simulink subsystem "Command_Data_handling"  (R2024a)
settings: Solver=VariableStepAuto  StartTime=0.0  StopTime=10.0  RelTol=1e-3
undefined symbols (not defined in the file): rfSatSourceSampleTime
libraries: simulink x1, commrandsrc3 x1
settings Model: Creator=dani  LastModifiedBy=dani

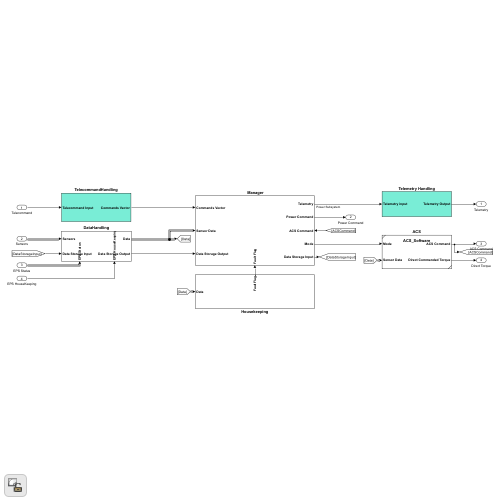
[thumbnail: Simulink's stored preview of the top-level diagram]
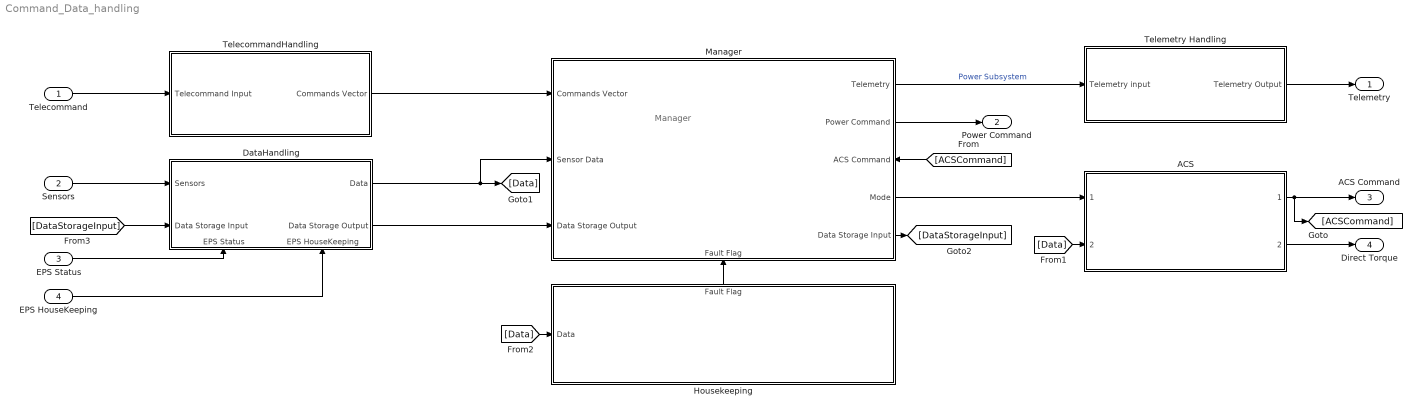
== system Command_Data_handling ==
  note: Manager
  Telecommand : Inport
  Sensors : Inport  Port=2
  EPS Status : Inport  Port=3
  EPS HouseKeeping : Inport  Port=4
  " Manager" : Subsystem
      settings: PortSchema="{\"entries\":[{\"content\":{\"sides\":[{\"content\":{\"connectorIds\":[\"In1\",\"In2\",\"In3\"]},\"type\":\"ConnectorPlacement.EquallySpacedRectSide\",\"uuid\":\"ec07d368-8191-42e4-9375-c2c602df22cf\"},{\"content\":{\"connectorIds\":[\"Out1\",\"Out2\",\"In5\",\"Out3\",\"Out4\"],\"side\":\"RIGHT\"},\"type\":\"ConnectorPlacement.EquallySpacedRectSide\",\"uuid\":\"bfabc2f5-2100-4bb6-919b-28e5c4a4cd4f\"},{\"content\":{\"side\":\"TOP\"},\"type\":\"ConnectorPlacement.EquallySpacedRectSide\",\"uuid\":\"1116e096-0190-44f1-9e3d-e2304f4178f6\"},{\"content\":{\"connectorIds\":[\"In4\"],\"side\":\"BOTTOM\"},\"type\":\"ConnectorPlacement.EquallySpacedRectSide\",\"uuid\":\"3d921d5d-5d93-4419-baa2-2f36ac6a4a99\"}]},\"type\":\"ConnectorPlacement.EquallySpacedConnector\",\"uuid\":\"03acd5cc-f7c7-46e5-a21e-c8fb7c082571\"}],\"packageUris\":[\"http://schema.mathworks.com/mf0/Connector/R2020b\"],\"version\":\"1.0\"}"
  ACS : Subsystem  ReferencedSubsystem=ACS_Software
  DataHandling : Subsystem
      settings: PortSchema="{\"entries\":[{\"content\":{\"sides\":[{\"content\":{\"connectorIds\":[\"In1\",\"In2\"]},\"type\":\"ConnectorPlacement.EquallySpacedRectSide\",\"uuid\":\"333a63f6-0788-485d-a40f-b2eefd028988\"},{\"content\":{\"connectorIds\":[\"Out1\",\"Out2\"],\"side\":\"RIGHT\"},\"type\":\"ConnectorPlacement.EquallySpacedRectSide\",\"uuid\":\"78b8a504-3dff-4f2b-a0ec-fa2bfb715213\"},{\"content\":{\"side\":\"TOP\"},\"type\":\"ConnectorPlacement.EquallySpacedRectSide\",\"uuid\":\"ac4bbea7-d5e7-4844-aab9-f621cfd7c534\"},{\"content\":{\"connectorIds\":[\"In3\",\"In4\"],\"side\":\"BOTTOM\"},\"type\":\"ConnectorPlacement.EquallySpacedRectSide\",\"uuid\":\"8bcb476b-069e-40da-9a40-a3d9d3480925\"}]},\"type\":\"ConnectorPlacement.EquallySpacedConnector\",\"uuid\":\"bbb35b76-fa73-457a-a216-c7062a4ce149\"}],\"packageUris\":[\"http://schema.mathworks.com/mf0/Connector/R2020b\"],\"version\":\"1.0\"}"
  Housekeeping : Subsystem
      settings: PortSchema="{\"entries\":[{\"content\":{\"sides\":[{\"content\":{\"connectorIds\":[\"In1\"]},\"type\":\"ConnectorPlacement.EquallySpacedRectSide\",\"uuid\":\"8eabc5dd-b460-4602-97d0-241e39b04916\"},{\"content\":{\"side\":\"RIGHT\"},\"type\":\"ConnectorPlacement.EquallySpacedRectSide\",\"uuid\":\"34fc1683-6b23-42e6-b522-0d805f5ee3a0\"},{\"content\":{\"connectorIds\":[\"Out1\"],\"side\":\"TOP\"},\"type\":\"ConnectorPlacement.EquallySpacedRectSide\",\"uuid\":\"2e5f843e-dd0f-45a3-97ce-c55e6bc4c9fd\"}]},\"type\":\"ConnectorPlacement.EquallySpacedConnector\",\"uuid\":\"4787b5c4-2ae8-477e-a21f-abe35d36bbd4\"}],\"packageUris\":[\"http://schema.mathworks.com/mf0/Connector/R2020b\"],\"version\":\"1.0\"}"
  TelecommandHandling : Subsystem
  Telemetry Handling : Subsystem
  Telemetry : Outport
  Power Command : Outport  Port=2
  ACS Command : Outport  Port=3
  Direct Torque : Outport  Port=4
  wires:
  " Manager"/1(Telemetry) -> Telemetry Handling/1(Telemetry input)  "Power Subsystem"
  Telecommand/1 -> TelecommandHandling/1(Telecommand Input)
  DataHandling/1(Data) -> [Data], " Manager"/2(Sensor Data)
  TelecommandHandling/1(Commands Vector) -> " Manager"/1(Commands Vector)
  Housekeeping/1(Fault Flag) -> " Manager"/4(Fault Flag)
  " Manager"/2(Power Command) -> Power Command/1
  Telemetry Handling/1(Telemetry Output) -> Telemetry/1
  Sensors/1 -> DataHandling/1(Sensors)
  DataHandling/2(Data Storage Output) -> " Manager"/3(Data Storage Output)
  " Manager"/3(Mode) -> ACS/1
  ACS/1 -> ACS Command/1, [ACSCommand]
  [ACSCommand] -> " Manager"/5(ACS Command)
  [Data] -> ACS/2
  [Data] -> Housekeeping/1("Data ")
  " Manager"/4(Data Storage Input) -> [DataStorageInput]
  [DataStorageInput] -> DataHandling/2(Data Storage Input)
  EPS Status/1 -> DataHandling/3(EPS Status)
  EPS HouseKeeping/1 -> DataHandling/4(EPS HouseKeeping)
  ACS/2 -> Direct Torque/1

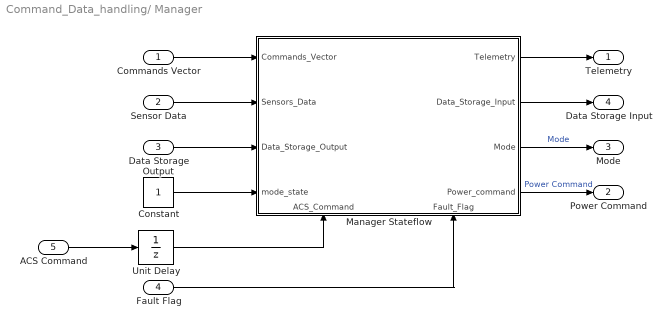
== system Command_Data_handling/ Manager ==
  Commands Vector : Inport
  Sensor Data : Inport  Port=2
  Data Storage Output : Inport  Port=3
  Fault Flag : Inport  Port=4
  ACS Command : Inport  Port=5
  Constant : Constant
  Manager Stateflow : Stateflow chart  TreatAsAtomicUnit=on
      settings: PortSchema="{\"entries\":[{\"content\":{\"sides\":[{\"content\":{\"connectorIds\":[\"In3\",\"In4\",\"In5\",\"In6\"]},\"type\":\"ConnectorPlacement.EquallySpacedRectSide\",\"uuid\":\"e1f10b30-4f11-427f-80a1-99253ceb8573\"},{\"content\":{\"connectorIds\":[\"Out1\",\"Out3\",\"Out4\",\"Out2\"],\"side\":\"RIGHT\"},\"type\":\"ConnectorPlacement.EquallySpacedRectSide\",\"uuid\":\"4c8c458e-9418-464f-accf-2ac8778338cd\"},{\"content\":{\"side\":\"TOP\"},\"type\":\"ConnectorPlacement.EquallySpacedRectSide\",\"uuid\":\"e00657ff-7d3d-45d1-9d17-1dfc8ef8ce11\"},{\"content\":{\"connectorIds\":[\"In1\",\"In2\"],\"side\":\"BOTTOM\"},\"type\":\"ConnectorPlacement.EquallySpacedRectSide\",\"uuid\":\"427faea7-f341-40f5-a655-462f7a6a3110\"}]},\"type\":\"ConnectorPlacement.EquallySpacedConnector\",\"uuid\":\"4ecfb0d2-db40-4a9e-b203-98a08a8aa01e\"}],\"packageUris\":[\"http://schema.mathworks.com/mf0/Connector/R2020b\"],\"version\":\"1.0\"}"
  Unit Delay : UnitDelay  SampleTime=-1  HasFrameUpgradeWarning=on
  Telemetry : Outport
  Power Command : Outport  Port=2
  Mode : Outport  Port=3
  Data Storage Input : Outport  Port=4
  wires:
  Manager Stateflow/3(Data_Storage_Input) -> Data Storage Input/1
  Manager Stateflow/4(Mode) -> Mode/1  "Mode"
  Fault Flag/1 -> Manager Stateflow/2(Fault_Flag)
  Constant/1 -> Manager Stateflow/6(mode_state)
  Unit Delay/1 -> Manager Stateflow/1(ACS_Command)
  Data Storage Output/1 -> Manager Stateflow/5(Data_Storage_Output)
  Sensor Data/1 -> Manager Stateflow/4(Sensors_Data)
  Manager Stateflow/1(Telemetry) -> Telemetry/1
  Manager Stateflow/2(Power_command) -> Power Command/1  "Power Command"
  Commands Vector/1 -> Manager Stateflow/3(Commands_Vector)
  ACS Command/1 -> Unit Delay/1

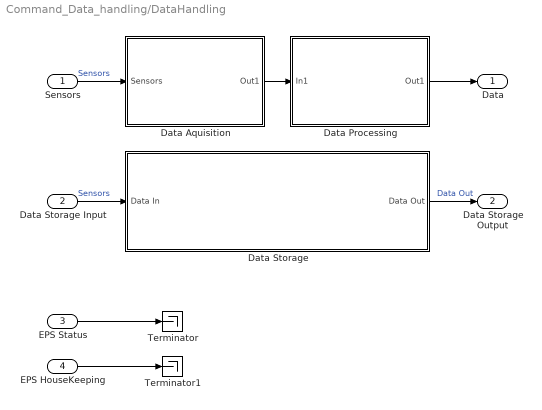
== system Command_Data_handling/DataHandling ==
  Sensors : Inport
  Data Storage Input : Inport  Port=2
  EPS Status : Inport  Port=3
  EPS HouseKeeping : Inport  Port=4
  Data Aquisition : Subsystem
  Data Processing : Subsystem
  Data Storage : Subsystem
  Terminator : Terminator
  Terminator1 : Terminator
  Data : Outport
  Data Storage Output : Outport  Port=2
  wires:
  EPS HouseKeeping/1 -> Terminator1/1
  EPS Status/1 -> Terminator/1
  Data Storage Input/1 -> Data Storage/1(Data In)  "Sensors"
  Data Processing/1(Out1) -> Data/1
  Data Storage/1(Data Out) -> Data Storage Output/1  "Data Out"
  Sensors/1 -> Data Aquisition/1(Sensors)  "Sensors"
  Data Aquisition/1(Out1) -> Data Processing/1(In1)

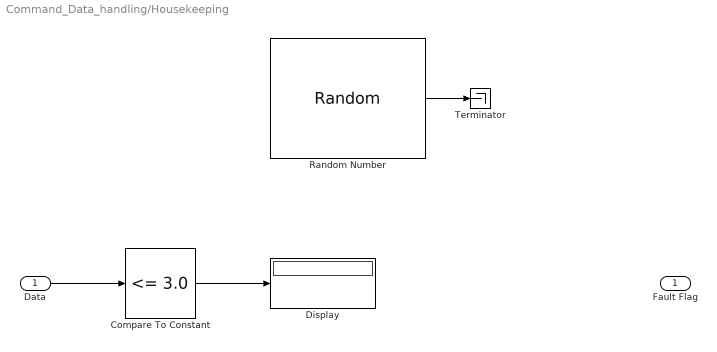
== system Command_Data_handling/Housekeeping ==
  "Data " : Inport
  Compare To Constant : simulink/Logic and Bit Operations/Compare To Constant  relop=<=  const=3.0  OutDataTypeStr=boolean
  Display : Display
  Random Number : RandomNumber  SampleTime=100
  Terminator : Terminator
  Fault Flag : Outport
  wires:
  Random Number/1 -> Terminator/1
  Compare To Constant/1 -> Display/1
  "Data "/1 -> Compare To Constant/1

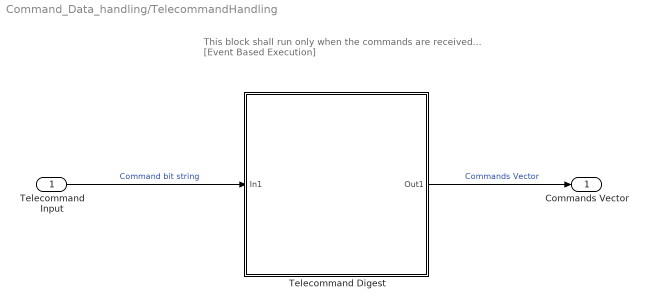
== system Command_Data_handling/TelecommandHandling ==
  note: This block shall run only when the commands
      |  are received... [Event Based Execution]
  Telecommand Input : Inport
  Telecommand Digest : Subsystem
  Commands Vector : Outport
  wires:
  Telecommand Digest/1(Out1) -> Commands Vector/1  "Commands Vector"
  Telecommand Input/1 -> Telecommand Digest/1(In1)  "Command bit string"

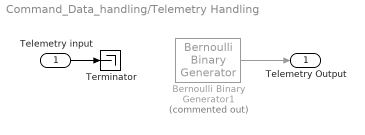
== system Command_Data_handling/Telemetry Handling ==
  Telemetry input : Inport
  Bernoulli Binary Generator1 : commrandsrc3/Bernoulli Binary Generator  Commented=on  ProbabilityOfZero=0.5  SeedSource=Parameter  Seed=37  SampleTime=rfSatSourceSampleTime  SamplesPerFrame=rfSatSourceSamplesPerSymbol  OutputDataType=double  SimulateUsing=Interpreted execution
  Terminator : Terminator
  Telemetry Output : Outport
  wires:
  Telemetry input/1 -> Terminator/1
  Bernoulli Binary Generator1/1 -> Telemetry Output/1

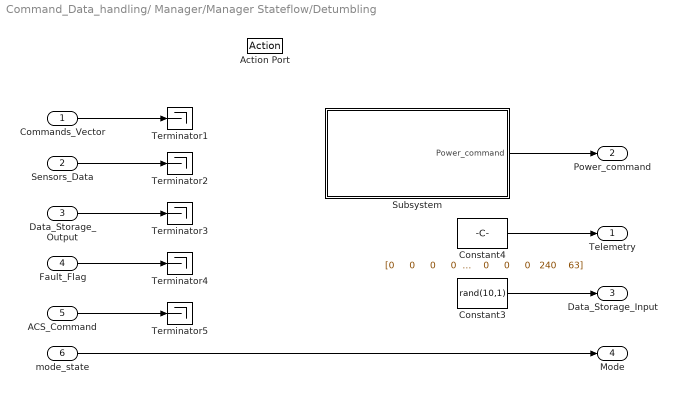
== system Command_Data_handling/ Manager/Manager Stateflow/Detumbling ==
  Commands_Vector : Inport
  Sensors_Data : Inport  Port=2
  Data_Storage_Output : Inport  Port=3
  Fault_Flag : Inport  Port=4
  ACS_Command : Inport  Port=5
  mode_state : Inport  Port=6
  Action Port : ActionPort
      settings: CopyFcn=Stateflow.SLINSF.SimulinkMan.removeBlockPreDeleteFcn  PreDeleteFcn=Stateflow.SLINSF.SimulinkMan.unsafePredeleteFcn
  Constant3 : Constant  Value=rand(10,1)
  Constant4 : Constant  Value="[0     0     0     0     0     0   240    63     0     0     0     0     0     0     0     0     0     0     0     0 0     0     0     0     0     0     0     0     0     0     0     0     0     0     0     0     0     0   240    63]"  OutDataTypeStr=uint8
  Subsystem : Subsystem
  Terminator{1..5} (5 alike) : Terminator
  Telemetry : Outport
  Power_command : Outport  Port=2
  Data_Storage_Input : Outport  Port=3
  Mode : Outport  Port=4
  wires:
  Subsystem/1(Power_command) -> Power_command/1
  mode_state/1 -> Mode/1
  ACS_Command/1 -> Terminator5/1
  Fault_Flag/1 -> Terminator4/1
  Constant3/1 -> Data_Storage_Input/1
  Constant4/1 -> Telemetry/1
  Data_Storage_Output/1 -> Terminator3/1
  Sensors_Data/1 -> Terminator2/1
  Commands_Vector/1 -> Terminator1/1

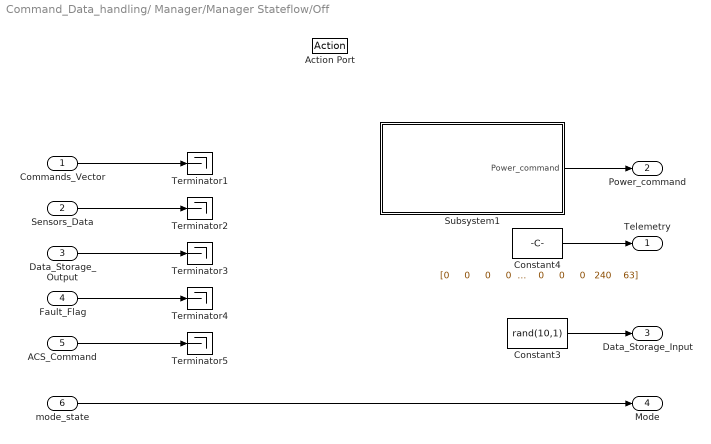
== system Command_Data_handling/ Manager/Manager Stateflow/Off ==
  Commands_Vector : Inport
  Sensors_Data : Inport  Port=2
  Data_Storage_Output : Inport  Port=3
  Fault_Flag : Inport  Port=4
  ACS_Command : Inport  Port=5
  mode_state : Inport  Port=6
  Action Port : ActionPort
      settings: CopyFcn=Stateflow.SLINSF.SimulinkMan.removeBlockPreDeleteFcn  PreDeleteFcn=Stateflow.SLINSF.SimulinkMan.unsafePredeleteFcn
  Constant3 : Constant  Value=rand(10,1)
  Constant4 : Constant  Value="[0     0     0     0     0     0   240    63     0     0     0     0     0     0     0     0     0     0     0     0 0     0     0     0     0     0     0     0     0     0     0     0     0     0     0     0     0     0   240    63]"  OutDataTypeStr=uint8
  Subsystem1 : Subsystem
  Terminator{1..5} (5 alike) : Terminator
  Telemetry : Outport
  Power_command : Outport  Port=2
  Data_Storage_Input : Outport  Port=3
  Mode : Outport  Port=4
  wires:
  mode_state/1 -> Mode/1
  ACS_Command/1 -> Terminator5/1
  Fault_Flag/1 -> Terminator4/1
  Constant3/1 -> Data_Storage_Input/1
  Subsystem1/1(Power_command) -> Power_command/1
  Constant4/1 -> Telemetry/1
  Data_Storage_Output/1 -> Terminator3/1
  Sensors_Data/1 -> Terminator2/1
  Commands_Vector/1 -> Terminator1/1

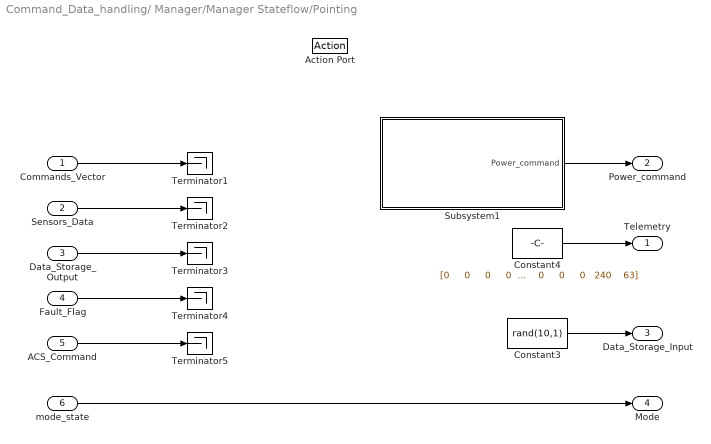
== system Command_Data_handling/ Manager/Manager Stateflow/Pointing ==
  Commands_Vector : Inport
  Sensors_Data : Inport  Port=2
  Data_Storage_Output : Inport  Port=3
  Fault_Flag : Inport  Port=4
  ACS_Command : Inport  Port=5
  mode_state : Inport  Port=6
  Action Port : ActionPort
      settings: CopyFcn=Stateflow.SLINSF.SimulinkMan.removeBlockPreDeleteFcn  PreDeleteFcn=Stateflow.SLINSF.SimulinkMan.unsafePredeleteFcn
  Constant3 : Constant  Value=rand(10,1)
  Constant4 : Constant  Value="[0     0     0     0     0     0   240    63     0     0     0     0     0     0     0     0     0     0     0     0 0     0     0     0     0     0     0     0     0     0     0     0     0     0     0     0     0     0   240    63]"  OutDataTypeStr=uint8
  Subsystem1 : Subsystem
  Terminator{1..5} (5 alike) : Terminator
  Telemetry : Outport
  Power_command : Outport  Port=2
  Data_Storage_Input : Outport  Port=3
  Mode : Outport  Port=4
  wires:
  mode_state/1 -> Mode/1
  ACS_Command/1 -> Terminator5/1
  Fault_Flag/1 -> Terminator4/1
  Constant3/1 -> Data_Storage_Input/1
  Subsystem1/1(Power_command) -> Power_command/1
  Constant4/1 -> Telemetry/1
  Data_Storage_Output/1 -> Terminator3/1
  Sensors_Data/1 -> Terminator2/1
  Commands_Vector/1 -> Terminator1/1

== system Command_Data_handling/DataHandling/Data Aquisition ==
  Sensors : Inport
  Out1 : Outport
  wires:
  Sensors/1 -> Out1/1

== system Command_Data_handling/DataHandling/Data Processing ==
  In1 : Inport
  Out1 : Outport
  wires:
  In1/1 -> Out1/1

== system Command_Data_handling/DataHandling/Data Storage ==
  Data In : Inport
  Delay : Delay
  Data Out : Outport
  wires:
  Delay/1 -> Data Out/1
  Data In/1 -> Delay/1

== system Command_Data_handling/TelecommandHandling/Telecommand Digest ==
  In1 : Inport
  Out1 : Outport
  wires:
  In1/1 -> Out1/1

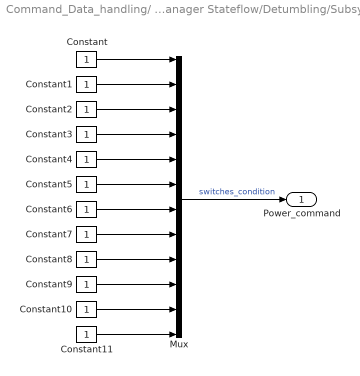
== system Command_Data_handling/ Manager/Manager Stateflow/Detumbling/Subsystem ==
  Constant{,1..11} (12 alike) : Constant
  Mux : Mux  Inputs=12
  Power_command : Outport
  wires:
  Constant6/1 -> Mux/7
  Constant7/1 -> Mux/8
  Constant8/1 -> Mux/9
  Constant9/1 -> Mux/10
  Constant10/1 -> Mux/11
  Constant11/1 -> Mux/12
  Constant5/1 -> Mux/6
  Constant4/1 -> Mux/5
  Constant3/1 -> Mux/4
  Constant2/1 -> Mux/3
  Constant1/1 -> Mux/2
  Mux/1 -> Power_command/1  "switches_condition"
  Constant/1 -> Mux/1

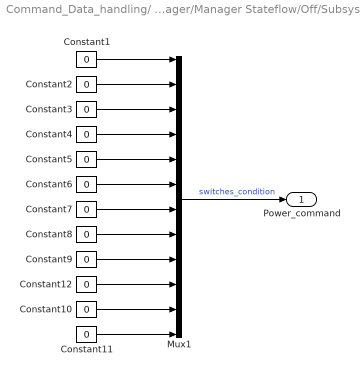
== system Command_Data_handling/ Manager/Manager Stateflow/Off/Subsystem1 ==
  Constant{1..12} (12 alike) : Constant  Value=0
  Mux1 : Mux  Inputs=12
  Power_command : Outport
  wires:
  Constant11/1 -> Mux1/12
  Constant12/1 -> Mux1/10
  Constant5/1 -> Mux1/5
  Constant2/1 -> Mux1/2
  Constant6/1 -> Mux1/6
  Mux1/1 -> Power_command/1  "switches_condition"
  Constant4/1 -> Mux1/4
  Constant1/1 -> Mux1/1
  Constant8/1 -> Mux1/8
  Constant7/1 -> Mux1/7
  Constant9/1 -> Mux1/9
  Constant10/1 -> Mux1/11
  Constant3/1 -> Mux1/3

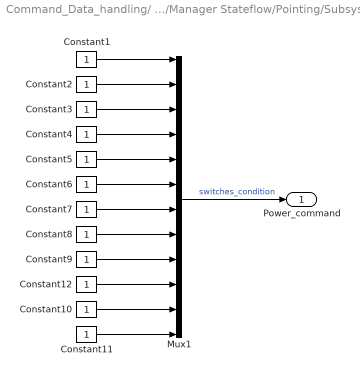
== system Command_Data_handling/ Manager/Manager Stateflow/Pointing/Subsystem1 ==
  Constant{1..12} (12 alike) : Constant
  Mux1 : Mux  Inputs=12
  Power_command : Outport
  wires:
  Constant11/1 -> Mux1/12
  Constant12/1 -> Mux1/10
  Constant5/1 -> Mux1/5
  Constant2/1 -> Mux1/2
  Constant6/1 -> Mux1/6
  Mux1/1 -> Power_command/1  "switches_condition"
  Constant4/1 -> Mux1/4
  Constant1/1 -> Mux1/1
  Constant8/1 -> Mux1/8
  Constant7/1 -> Mux1/7
  Constant9/1 -> Mux1/9
  Constant10/1 -> Mux1/11
  Constant3/1 -> Mux1/3

== stateflow chart Command_Data_handling/ Manager/Manager Stateflow ==
  state Off
  state Pointing
  state Detumbling
  state Boot
    mode_state;
  Boot -> Off [order 3] : [mode_state == 0]
  Boot -> Pointing [order 2] : [mode_state == 2]
  Boot -> Detumbling [order 1] : [mode_state == 1]
  (default) -> Boot
  data: sf_internal_action_state_placeholder_data local double size=1 =0; sf_internal_action_state_placeholder_data local double size=1 =0; sf_internal_action_state_placeholder_data local double size=1 =0; ACS_Command input; Fault_Flag input; Commands_Vector input; Sensors_Data input; Data_Storage_Output input; Telemetry output; Power_command output; Data_Storage_Input output; Mode output; mode_state input double
